simulink model "q1_a"  (R2026a)
settings: Solver=VariableStepAuto
model workspace (MAT data in the model file):
  K = Simulink.Parameter
  K.Value = 1
  K.Complexity = 'real'
  K.Dimensions = [1 1]
  K.DataType = 'auto'
  a = Simulink.Parameter
  a.Value = 2
  a.Complexity = 'real'
  a.Dimensions = [1 1]
  a.DataType = 'auto'
  k = 5
  k1 = Simulink.Parameter
  k1.Value = 4
  k1.Complexity = 'real'
  k1.Dimensions = [1 1]
  k1.DataType = 'auto'
  k2 = Simulink.Parameter
  k2.Value = 6
  k2.Complexity = 'real'
  k2.Dimensions = [1 1]
  k2.DataType = 'auto'
values from neighbouring files (symbols this model uses):
  k1 = wc^2    (= 1)    [q2.m]
  k2 = 2*zc*wc - gamma*wc^2    (= 0.914)    [q2.m]
settings Model: Creator=LAB_PC  LastModifiedBy=LAB_PC

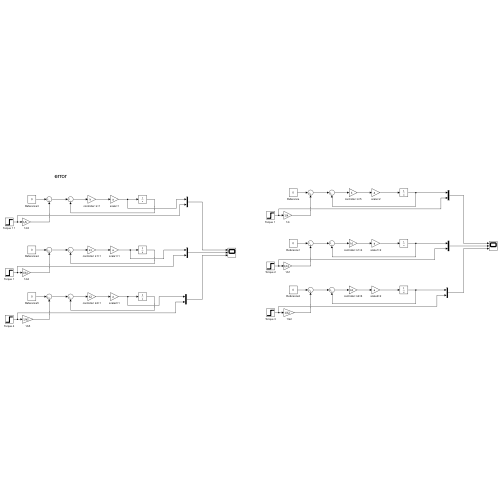
[thumbnail: Simulink's stored preview of the top-level diagram]
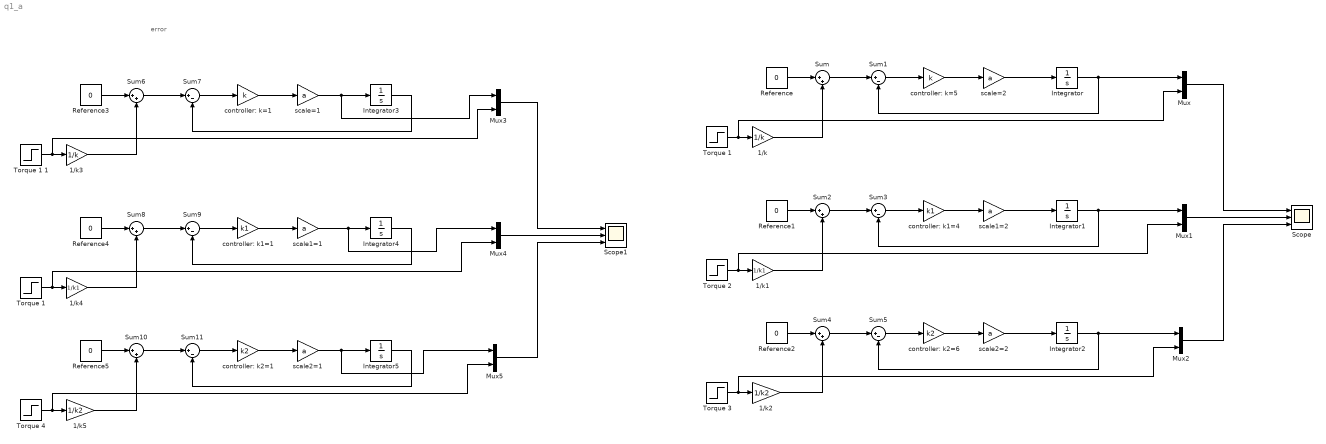
== system q1_a ==
  note: error
  1/k : Gain  Gain=1/k
  1/k1 : Gain  Gain=1/k1
  1/k2 : Gain  Gain=1/k2
  1/k3 : Gain  Gain=1/k
  1/k4 : Gain  Gain=1/k1
  1/k5 : Gain  Gain=1/k2
  Integrator{,1..5} (6 alike) : Integrator
  Mux{,1..5} (6 alike) : Mux  Inputs=2
  Reference{,1..5} (6 alike) : Constant  Value=0
  Scope : Scope  NumInputPorts=3
      settings: TimeAxisLabels=None  ActiveDisplayYMinimum=-0.27459016393442637  ActiveDisplayYMaximum=2.3504098360655741  DataLoggingVariableName=ScopeData2
  Scope1 : Scope  NumInputPorts=3
      settings: TimeAxisLabels=None  ActiveDisplayYMinimum=-0.27459016393442637  ActiveDisplayYMaximum=2.3504098360655741
  Sum{,2,4,6,8,10} (6 alike) : Sum  Inputs=|++
  Sum{1,3,5,7,9,11} (6 alike) : Sum  Inputs=|+-
  Torque {1..4} (4 alike) : Step  SampleTime=0
  "Torque 1 " : Step  SampleTime=0
  Torque 1 1 : Step  SampleTime=0
  controller: k1=1 : Gain  Gain=k1
  controller: k1=4 : Gain  Gain=k1
  controller: k2=1 : Gain  Gain=k2
  controller: k2=6 : Gain  Gain=k2
  controller: k=1 : Gain  Gain=k
  controller: k=5 : Gain  Gain=k
  scale1=1 : Gain  Gain=a
  scale1=2 : Gain  Gain=a
  scale2=1 : Gain  Gain=a
  scale2=2 : Gain  Gain=a
  scale=1 : Gain  Gain=a
  scale=2 : Gain  Gain=a
  wires:
  controller: k=5/1 -> scale=2/1
  scale=2/1 -> Integrator/1
  Sum1/1 -> controller: k=5/1
  Reference/1 -> Sum/1
  1/k/1 -> Sum/2
  "Torque 1 "/1 -> Mux/2, 1/k/1
  Sum/1 -> Sum1/1
  Integrator/1 -> Sum1/2, Mux/1
  controller: k1=4/1 -> scale1=2/1
  1/k1/1 -> Sum2/2
  Torque 2/1 -> Mux1/2, 1/k1/1
  Reference1/1 -> Sum2/1
  Sum3/1 -> controller: k1=4/1
  Sum2/1 -> Sum3/1
  scale1=2/1 -> Integrator1/1
  Integrator1/1 -> Sum3/2, Mux1/1
  Integrator2/1 -> Mux2/1, Sum5/2
  scale2=2/1 -> Integrator2/1
  Sum4/1 -> Sum5/1
  controller: k2=6/1 -> scale2=2/1
  Sum5/1 -> controller: k2=6/1
  1/k2/1 -> Sum4/2
  Reference2/1 -> Sum4/1
  Torque 3/1 -> Mux2/2, 1/k2/1
  Mux/1 -> Scope/1
  Mux1/1 -> Scope/2
  Mux2/1 -> Scope/3
  controller: k=1/1 -> scale=1/1
  Mux5/1 -> Scope1/3
  Torque 1 1/1 -> Mux3/2, 1/k3/1
  1/k5/1 -> Sum10/2
  scale1=1/1 -> Mux4/1, Integrator4/1
  Sum7/1 -> controller: k=1/1
  Sum9/1 -> controller: k1=1/1
  Sum10/1 -> Sum11/1
  Torque 1/1 -> Mux4/2, 1/k4/1
  Sum6/1 -> Sum7/1
  Torque 4/1 -> Mux5/2, 1/k5/1
  Reference4/1 -> Sum8/1
  Sum8/1 -> Sum9/1
  1/k3/1 -> Sum6/2
  Sum11/1 -> controller: k2=1/1
  Reference5/1 -> Sum10/1
  Integrator4/1 -> Sum9/2
  Integrator5/1 -> Sum11/2
  Mux4/1 -> Scope1/2
  controller: k2=1/1 -> scale2=1/1
  Mux3/1 -> Scope1/1
  Integrator3/1 -> Sum7/2
  scale2=1/1 -> Mux5/1, Integrator5/1
  scale=1/1 -> Mux3/1, Integrator3/1
  Reference3/1 -> Sum6/1
  1/k4/1 -> Sum8/2
  controller: k1=1/1 -> scale1=1/1
